simulink model "LQRandPIDcontrollerForIP"  (R2014a)
settings: Solver=ode45  StartTime=0.0  StopTime=100  RelTol=1e-3
settings Model: Creator=ControlSystemLab  LastModifiedBy=MMMUT8
settings DebuggingCC: UnderspecifiedInitializationDetection=Classic  StateNameClashWarn=warning

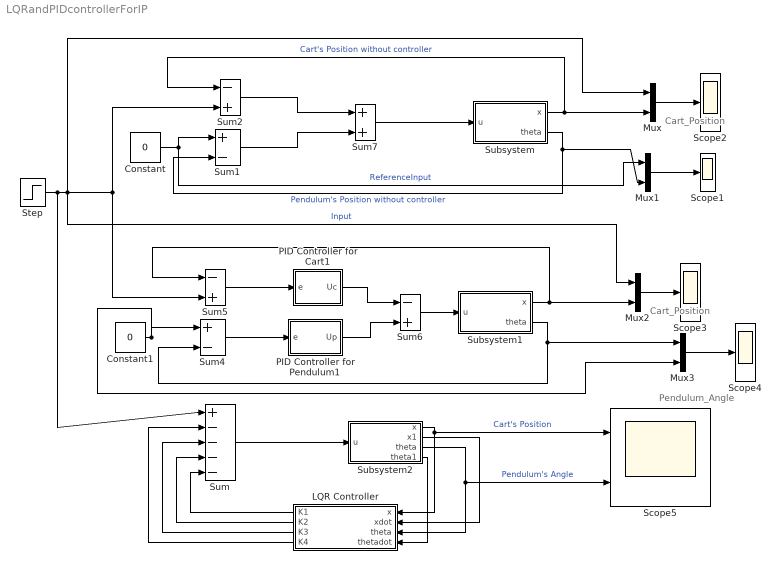
== system LQRandPIDcontrollerForIP ==
  note: Cart_Position
  note: Pendulum_Angle
  note: Cart_Position
  Constant : Constant  Value=0
  Constant1 : Constant  Value=0
  LQR Controller : Subsystem
  Mux{,1..3} (4 alike) : Mux  Inputs=2
  PID Controller for Cart1 : Subsystem
  PID Controller for Pendulum1 : Subsystem
  Scope{1..4} (4 alike) : Scope
      Scope1 settings: ShowLegends=on
      Scope2 settings: ShowLegends=on  TimeRange=100  YMin=-4.999999999999999e+105  YMax=4.5e+106
      Scope3 settings: ShowLegends=on  SaveName=ScopeData2
      Scope4 settings: ShowLegends=on  SaveName=ScopeData3
  Scope5 : Scope  NumInputPorts=2
      settings: ShowLegends=on  TimeRange=10  YMin=-5~-0.002  YMax=5~0.004  SaveName=LQR
  Step : Step  SampleTime=0
  Subsystem : Subsystem
  Subsystem1 : Subsystem
  Subsystem2 : Subsystem
  Sum : Sum  Inputs=|+----
  Sum1 : Sum  Inputs=|+-
  Sum2 : Sum  Inputs=-|+
  Sum4 : Sum  Inputs=|+-
  Sum5 : Sum  Inputs=-|+
  Sum6 : Sum  Inputs=-|+
  Sum7 : Sum
  wires:
  Sum/1 -> Subsystem2/1(u)
  Subsystem2/2(x1) -> LQR Controller/2(xdot)
  Subsystem2/4(theta1) -> LQR Controller/4(thetadot)
  LQR Controller/1(K1) -> Sum/5
  LQR Controller/2(K2) -> Sum/4
  LQR Controller/3(K3) -> Sum/3
  LQR Controller/4(K4) -> Sum/2
  Subsystem2/1(x) -> LQR Controller/1(x), Scope5/1  "Cart's Position"
  Subsystem2/3(theta) -> Scope5/2, LQR Controller/3(theta)  "Pendulum's Angle"
  Subsystem/1(x) -> Mux/2, Sum2/1  "Cart's Position without controller"
  Constant/1 -> Mux1/1, Sum1/1  "ReferenceInput"
  Mux/1 -> Scope2/1
  Step/1 -> Sum/1, Mux2/1, Mux/1, Sum2/2, Sum5/2  "Input"
  Sum6/1 -> Subsystem1/1(u)
  PID Controller for Cart1/1(Uc) -> Sum6/1
  PID Controller for Pendulum1/1(Up) -> Sum6/2
  Sum4/1 -> PID Controller for Pendulum1/1(e)
  Sum5/1 -> PID Controller for Cart1/1(e)
  Constant1/1 -> Mux3/2, Sum4/1
  Mux2/1 -> Scope3/1
  Subsystem1/2(theta) -> Mux3/1, Sum4/2
  Subsystem1/1(x) -> Mux2/2, Sum5/1
  Subsystem/2(theta) -> Mux1/2, Sum1/2  "Pendulum's Position without controller"
  Mux1/1 -> Scope1/1
  Mux3/1 -> Scope4/1
  Sum7/1 -> Subsystem/1(u)
  Sum2/1 -> Sum7/1
  Sum1/1 -> Sum7/2

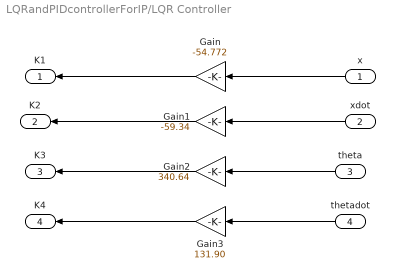
== system LQRandPIDcontrollerForIP/LQR Controller ==
  x : Inport
  xdot : Inport  Port=2
  theta : Inport  Port=3
  thetadot : Inport  Port=4
  Gain : Gain  Gain=-54.772
  Gain1 : Gain  Gain=-59.34
  Gain2 : Gain  Gain=340.64
  Gain3 : Gain  Gain=131.90
  K1 : Outport
  K2 : Outport  Port=2
  K3 : Outport  Port=3
  K4 : Outport  Port=4
  wires:
  x/1 -> Gain/1
  xdot/1 -> Gain1/1
  theta/1 -> Gain2/1
  thetadot/1 -> Gain3/1
  Gain/1 -> K1/1
  Gain1/1 -> K2/1
  Gain2/1 -> K3/1
  Gain3/1 -> K4/1

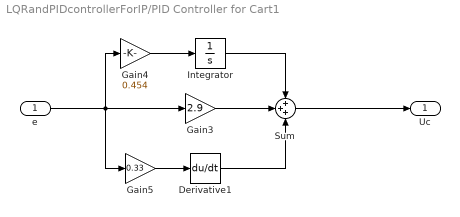
== system LQRandPIDcontrollerForIP/PID Controller for Cart1 ==
  e : Inport
  Derivative1 : Derivative
  Gain3 : Gain  Gain=2.9
  Gain4 : Gain  Gain=0.454
  Gain5 : Gain  Gain=0.33
  Integrator : Integrator
  Sum : Sum  Inputs=+++
  Uc : Outport
  wires:
  Gain5/1 -> Derivative1/1
  e/1 -> Gain4/1, Gain3/1, Gain5/1
  Sum/1 -> Uc/1
  Integrator/1 -> Sum/1
  Gain4/1 -> Integrator/1
  Gain3/1 -> Sum/2
  Derivative1/1 -> Sum/3

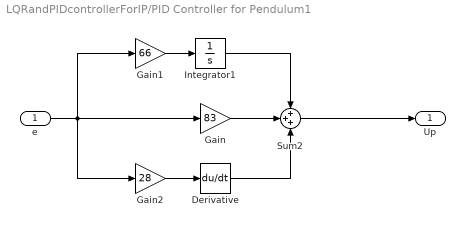
== system LQRandPIDcontrollerForIP/PID Controller for Pendulum1 ==
  e : Inport
  Derivative : Derivative
  Gain : Gain  Gain=83
  Gain1 : Gain  Gain=66
  Gain2 : Gain  Gain=28
  Integrator1 : Integrator
  Sum2 : Sum  Inputs=+++
  Up : Outport
  wires:
  Integrator1/1 -> Sum2/1
  Gain/1 -> Sum2/2
  Derivative/1 -> Sum2/3
  Gain1/1 -> Integrator1/1
  Gain2/1 -> Derivative/1
  e/1 -> Gain2/1, Gain1/1, Gain/1
  Sum2/1 -> Up/1

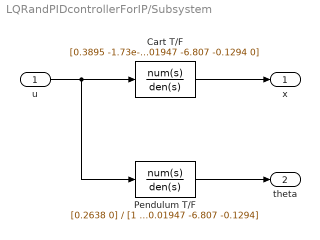
== system LQRandPIDcontrollerForIP/Subsystem ==
  u : Inport
  Cart T/F : TransferFcn  Numerator=[0.3895 -1.73e-16 -2.588]  Denominator=[1 0.01947 -6.807 -0.1294 0]
  Pendulum T/F : TransferFcn  Numerator=[0.2638 0]  Denominator=[1 0.01947 -6.807 -0.1294]
  x : Outport
  theta : Outport  Port=2
  wires:
  Cart T/F/1 -> x/1
  Pendulum T/F/1 -> theta/1
  u/1 -> Pendulum T/F/1, Cart T/F/1

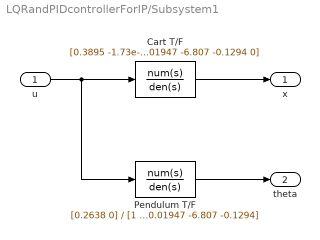
== system LQRandPIDcontrollerForIP/Subsystem1 ==
  u : Inport
  Cart T/F : TransferFcn  Numerator=[0.3895 -1.73e-16 -2.588]  Denominator=[1 0.01947 -6.807 -0.1294 0]
  Pendulum T/F : TransferFcn  Numerator=[0.2638 0]  Denominator=[1 0.01947 -6.807 -0.1294]
  x : Outport
  theta : Outport  Port=2
  wires:
  Cart T/F/1 -> x/1
  Pendulum T/F/1 -> theta/1
  u/1 -> Pendulum T/F/1, Cart T/F/1

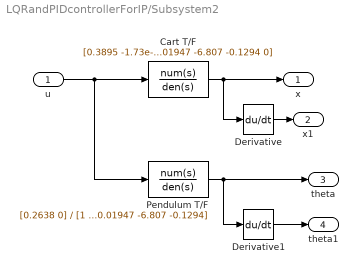
== system LQRandPIDcontrollerForIP/Subsystem2 ==
  u : Inport
  Cart T/F : TransferFcn  Numerator=[0.3895 -1.73e-16 -2.588]  Denominator=[1 0.01947 -6.807 -0.1294 0]
  Derivative : Derivative
  Derivative1 : Derivative
  Pendulum T/F : TransferFcn  Numerator=[0.2638 0]  Denominator=[1 0.01947 -6.807 -0.1294]
  x : Outport
  x1 : Outport  Port=2
  theta : Outport  Port=3
  theta1 : Outport  Port=4
  wires:
  Cart T/F/1 -> Derivative/1, x/1
  Pendulum T/F/1 -> theta/1, Derivative1/1
  u/1 -> Pendulum T/F/1, Cart T/F/1
  Derivative/1 -> x1/1
  Derivative1/1 -> theta1/1
